simulink model "LegoEV3_poursuite"  (R2025b)
settings: Solver=FixedStepAuto  StartTime=0.0  StopTime=10.0  RelTol=1e-3  EnableMultiTasking=on
values from neighbouring files (symbols this model uses):
  K_corr = acker(Ad,Bd,poles_souhaites)    [model.m]
  K_PWM = 8.087    [model.m]
  S_corr = inv([1 0 0 0]*inv(eye(4)-Ad+Bd*K_corr)*Bd)    [model.m]
  Ts = 0.004    [model.m]
undefined symbols (not defined in the file or in its folder): DiscIntNeverNeededParam, gamma
libraries: legoev3lib x8, simulink x1
settings Model: ExtModeTrigDuration=2  Creator=carol  LastModifiedBy=alber
settings SolverCC: PositivePriorityOrder=on
settings OptimizationCC: DefaultParameterBehavior=Inlined  EnhancedBackFolding=on  PassReuseOutputArgsAs=Individual arguments  ZeroExternalMemoryAtStartup=off  ZeroInternalMemoryAtStartup=off  MaxStackSize=64  OptimizeBlockOrder=speed  DifferentSizesBufferReuse=on  OptimizationCustomize=off  EfficientTunableParamExpr=on
settings DebuggingCC: ParameterTunabilityLossMsg=error
settings HardwareCC: ProdBitPerPointer=32.0  ProdBitPerSizeT=32.0  ProdBitPerPtrDiffT=32.0  ProdLargestAtomicInteger=Long  ProdWordSize=32.0  ProdHWDeviceType=ARM Compatible->ARM 9  UseEmbeddedCoderFeatures=off  UseSimulinkCoderFeatures=off
settings SFSimCC: MATLABDynamicMemAlloc=off
settings RTWCC: SystemTargetFile=ert.tlc  HardwareBoard=LEGO MINDSTORMS EV3  TLCOptions="-aInlineSetEventsForThisBaseRateFcn=TLC_FALSE -aSuppressMultiTaskScheduler=TLC_FALSE  -aRateBasedStepFcn=0"  TemplateMakefile=ert_default_tmf  Toolchain=Sourcery G++ Lite v2009q3  Description=Embedded Coder
settings CodeAppCC: ForceParamTrailComments=on  IgnoreCustomStorageClasses=off  OperatorAnnotations=on  SimulinkDataObjDesc=on  SFDataObjDesc=on  InsertBlockDesc=on
settings ERTTargetCC: ExtModeTransport=2.0  ExtModeStaticAlloc=on  ExtModeMexFile=ext_xcp  ExtModeIntrfLevel=Level2 - Open  SupportContinuousTime=on  SupportNonInlinedSFcns=on  SupportVariableSizeSignals=on

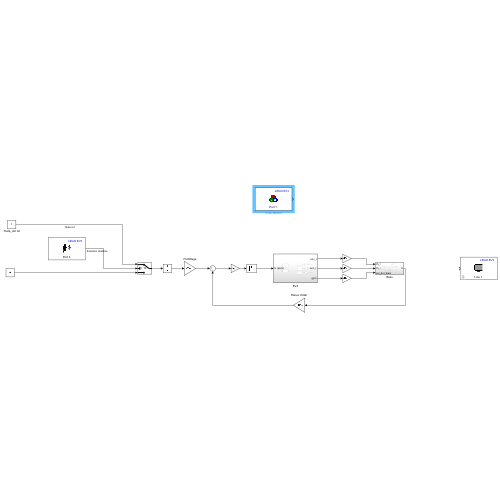
[thumbnail: Simulink's stored preview of the top-level diagram]
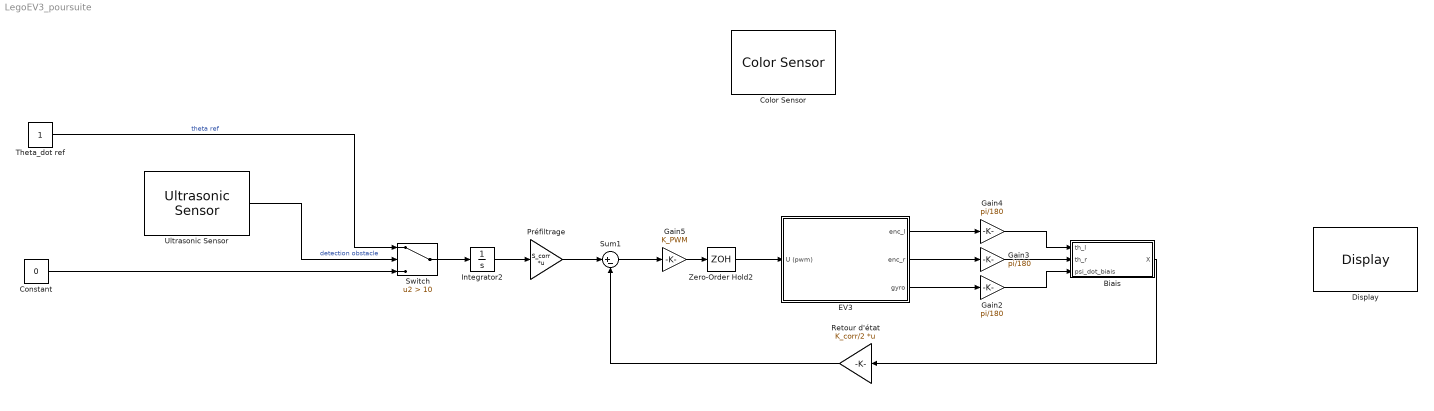
== system LegoEV3_poursuite ==
  Biais : Subsystem
  Color Sensor : legoev3lib/Color Sensor  portNumber=1  mode=Color  sampleTime=0.1
  Constant : Constant  Value=0
  Display : legoev3lib/Display  slcdLine=1  slcdFormat=Decimal
  EV3 : Subsystem
  Gain2 : Gain  Gain=pi/180
  Gain3 : Gain  Gain=pi/180
  Gain4 : Gain  Gain=pi/180
  Gain5 : Gain  Gain=K_PWM
  Integrator2 : Integrator
  Préfiltrage : Gain  Gain=S_corr  Multiplication=Matrix(K*u)
  Retour d'état : Gain  Gain=K_corr/2  Multiplication=Matrix(K*u)
  Sum1 : Sum  Inputs=|+-
  Switch : Switch  Criteria=u2 > Threshold  Threshold=10  SaturateOnIntegerOverflow=off  InputSameDT=off
  Theta_dot ref : Constant  SampleTime=Ts
  Ultrasonic Sensor : legoev3lib/Ultrasonic Sensor  PortNumber=4  sampleTime=Ts
  Zero-Order Hold2 : ZeroOrderHold  SampleTime=Ts
  wires:
  EV3/3(gyro) -> Gain2/1
  Gain4/1 -> Biais/1(th_l)
  Biais/1(X) -> Retour d'état/1
  EV3/1(enc_l) -> Gain4/1
  Gain3/1 -> Biais/2(th_r)
  Gain2/1 -> Biais/3(psi_dot_biais)
  EV3/2(enc_r) -> Gain3/1
  Sum1/1 -> Gain5/1
  Zero-Order Hold2/1 -> EV3/1(U (pwm))
  Préfiltrage/1 -> Sum1/1
  Gain5/1 -> Zero-Order Hold2/1
  Retour d'état/1 -> Sum1/2
  Theta_dot ref/1 -> Switch/1  "theta ref"
  Switch/1 -> Integrator2/1
  Ultrasonic Sensor/1 -> Switch/2  "detection obstacle"
  Constant/1 -> Switch/3
  Integrator2/1 -> Préfiltrage/1

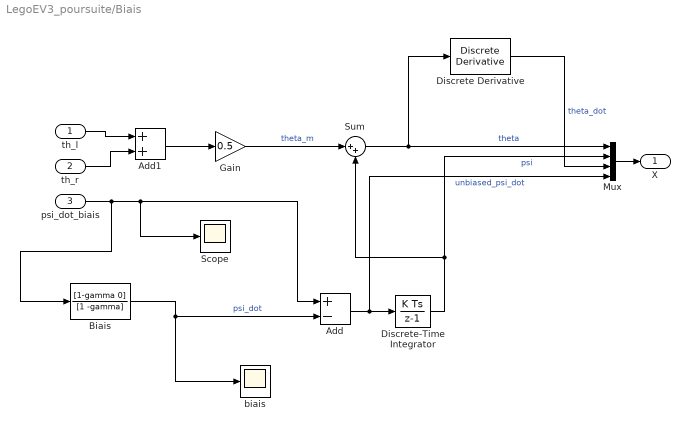
== system LegoEV3_poursuite/Biais ==
  th_l : Inport
  th_r : Inport  Port=2
  psi_dot_biais : Inport  Port=3
  Add : Sum  Inputs=+-
  Add1 : Sum
  Biais : DiscreteTransferFcn  Numerator=[1-gamma 0]  Denominator=[1 -gamma]
  Discrete Derivative : simulink/Quick Insert/Discrete/Discrete Derivative  gainval=1.0  ICPrevScaledInput=0.0  OutMin=[]  OutMax=[]  OutDataType=fixdt(1, 16)  OutScaling=2^-10  DoSatur=off
  Discrete-Time Integrator : DiscreteIntegrator  SampleTime=Ts  ICPrevOutput=DiscIntNeverNeededParam  ICPrevScaledInput=DiscIntNeverNeededParam
  Gain : Gain  Gain=0.5
  Mux : Mux
  Scope : Scope
      settings: ActiveDisplayYMinimum=-1  ActiveDisplayYMaximum=1  DataLoggingVariableName=ScopeData13
  Sum : Sum  Inputs=|++
  biais : Scope
      settings: ActiveDisplayYMinimum=-0.1164059395354744  ActiveDisplayYMaximum=0.0646369691442869  DataLoggingVariableName=ScopeData12
  X : Outport
  wires:
  th_l/1 -> Add1/1
  th_r/1 -> Add1/2
  Add1/1 -> Gain/1
  Mux/1 -> X/1
  Discrete Derivative/1 -> Mux/3  "theta_dot"
  Discrete-Time Integrator/1 -> Sum/2, Mux/2  "psi"
  psi_dot_biais/1 -> Biais/1, Scope/1, Add/1
  Biais/1 -> Add/2, biais/1  "psi_dot"
  Add/1 -> Mux/4, Discrete-Time Integrator/1  "unbiased_psi_dot"
  Gain/1 -> Sum/1  "theta_m"
  Sum/1 -> Mux/1, Discrete Derivative/1  "theta"

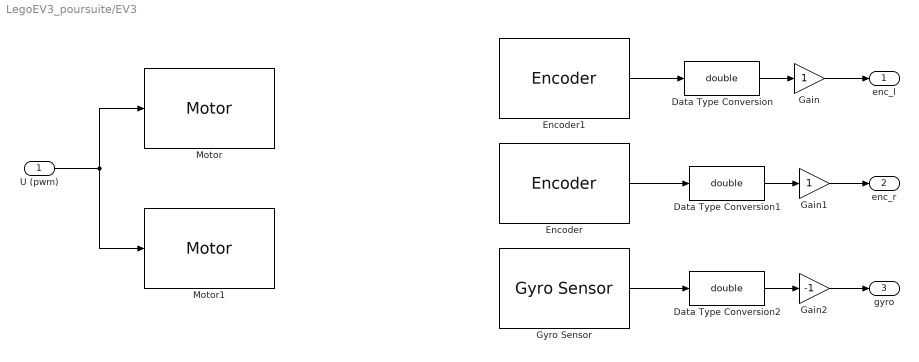
== system LegoEV3_poursuite/EV3 ==
  U (pwm) : Inport
  Data Type Conversion : DataTypeConversion  OutDataTypeStr=double  SaturateOnIntegerOverflow=off  RndMeth=Floor
  Data Type Conversion1 : DataTypeConversion  OutDataTypeStr=double  SaturateOnIntegerOverflow=off  RndMeth=Floor
  Data Type Conversion2 : DataTypeConversion  OutDataTypeStr=double  SaturateOnIntegerOverflow=off  RndMeth=Floor
  Encoder : legoev3lib/Encoder  portNumber=A  opMode=Reset by external signal  sampleTime=Ts
  Encoder1 : legoev3lib/Encoder  portNumber=D  opMode=Reset by external signal  sampleTime=Ts
  Gain : Gain
  Gain1 : Gain
  Gain2 : Gain  Gain=-1
  Gyro Sensor : legoev3lib/Gyro Sensor  portNumber=3  sampleTime=Ts
  Motor : legoev3lib/Motor  sportNumber=D  sstopAction=Brake
  Motor1 : legoev3lib/Motor  sportNumber=A  sstopAction=Brake
  enc_l : Outport
  enc_r : Outport  Port=2
  gyro : Outport  Port=3
  wires:
  Gyro Sensor/1 -> Data Type Conversion2/1
  Encoder/1 -> Data Type Conversion1/1
  Encoder1/1 -> Data Type Conversion/1
  Data Type Conversion/1 -> Gain/1
  Data Type Conversion1/1 -> Gain1/1
  Data Type Conversion2/1 -> Gain2/1
  U (pwm)/1 -> Motor1/1, Motor/1
  Gain/1 -> enc_l/1
  Gain1/1 -> enc_r/1
  Gain2/1 -> gyro/1
